simulink model "SimulareModel1"  (R2023a)
settings: Solver=VariableStepAuto  StartTime=0.0  StopTime=75.3  RelTol=1e-3
values from neighbouring files (symbols this model uses):
  Ts = 0.1    [NonLinearARXModel.mat]    (also in NonLinearHammerstein-Weiner.mat; Workspace.mat)
settings Model: Creator=petri  LastModifiedBy=petri

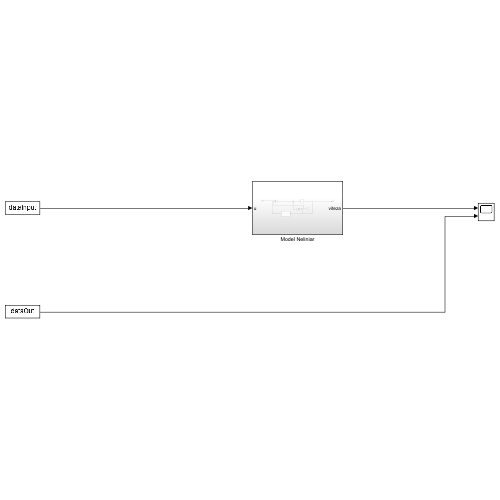
[thumbnail: Simulink's stored preview of the top-level diagram]
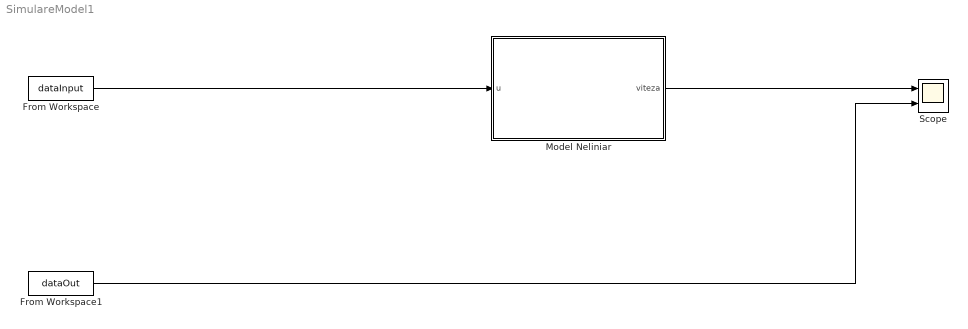
== system SimulareModel1 ==
  From Workspace : FromWorkspace  VariableName=dataInput  SampleTime=Ts
  From Workspace1 : FromWorkspace  VariableName=dataOut  SampleTime=Ts
  Model Neliniar : Subsystem
  Scope : Scope  NumInputPorts=2
  wires:
  From Workspace/1 -> Model Neliniar/1(u)
  Model Neliniar/1(viteza) -> Scope/1
  From Workspace1/1 -> Scope/2

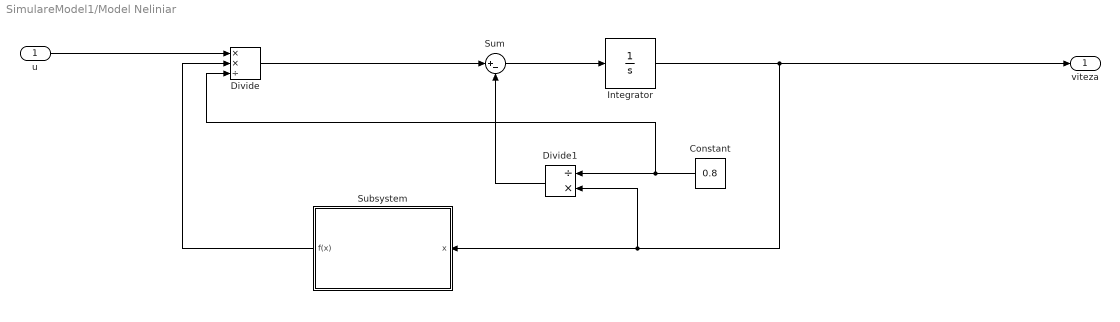
== system SimulareModel1/Model Neliniar ==
  u : Inport
  Constant : Constant  Value=0.8
  Divide : Product  Inputs=**/
  Divide1 : Product  Inputs=/*
  Integrator : Integrator
  Subsystem : Subsystem
  Sum : Sum  Inputs=|+-
  viteza : Outport
  wires:
  u/1 -> Divide/1
  Constant/1 -> Divide1/1, Divide/3
  Integrator/1 -> viteza/1, Subsystem/1(x), Divide1/2
  Sum/1 -> Integrator/1
  Divide1/1 -> Sum/2
  Divide/1 -> Sum/1
  Subsystem/1(f(x)) -> Divide/2

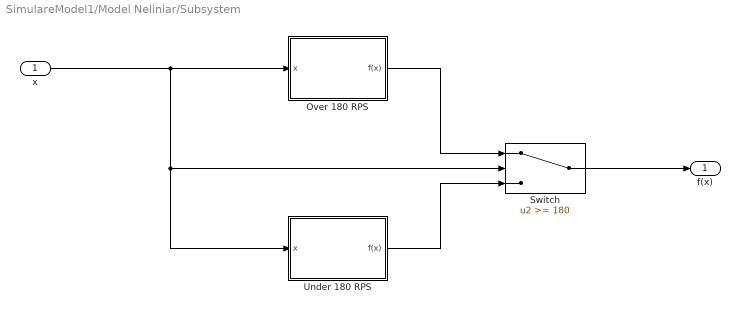
== system SimulareModel1/Model Neliniar/Subsystem ==
  x : Inport
  Over 180 RPS : Subsystem
  Switch : Switch  Threshold=180  SaturateOnIntegerOverflow=off  InputSameDT=off
  Under 180 RPS : Subsystem
  f(x) : Outport
  wires:
  x/1 -> Under 180 RPS/1(x), Switch/2, Over 180 RPS/1(x)
  Under 180 RPS/1(f(x)) -> Switch/3
  Over 180 RPS/1(f(x)) -> Switch/1
  Switch/1 -> f(x)/1

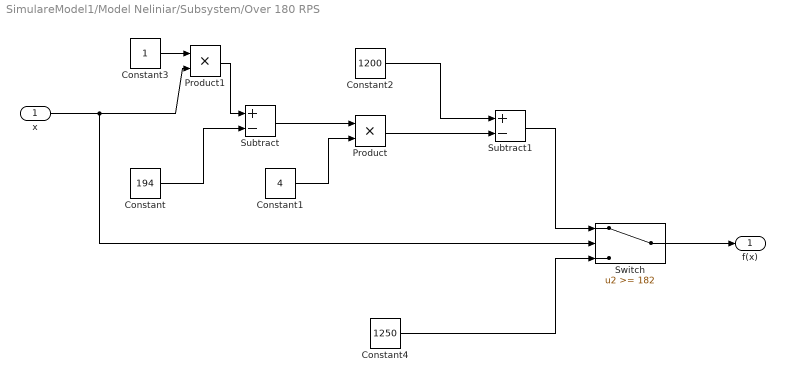
== system SimulareModel1/Model Neliniar/Subsystem/Over 180 RPS ==
  x : Inport
  Constant : Constant  Value=194  VectorParams1D=off
  Constant1 : Constant  Value=4
  Constant2 : Constant  Value=1200
  Constant3 : Constant
  Constant4 : Constant  Value=1250
  Product : Product
  Product1 : Product
  Subtract : Sum  Inputs=+-
  Subtract1 : Sum  Inputs=+-
  Switch : Switch  Threshold=182  SaturateOnIntegerOverflow=off  InputSameDT=off
  f(x) : Outport
  wires:
  x/1 -> Product1/2, Switch/2
  Product/1 -> Subtract1/2
  Constant3/1 -> Product1/1
  Constant/1 -> Subtract/2
  Subtract/1 -> Product/1
  Product1/1 -> Subtract/1
  Constant1/1 -> Product/2
  Constant2/1 -> Subtract1/1
  Constant4/1 -> Switch/3
  Subtract1/1 -> Switch/1
  Switch/1 -> f(x)/1

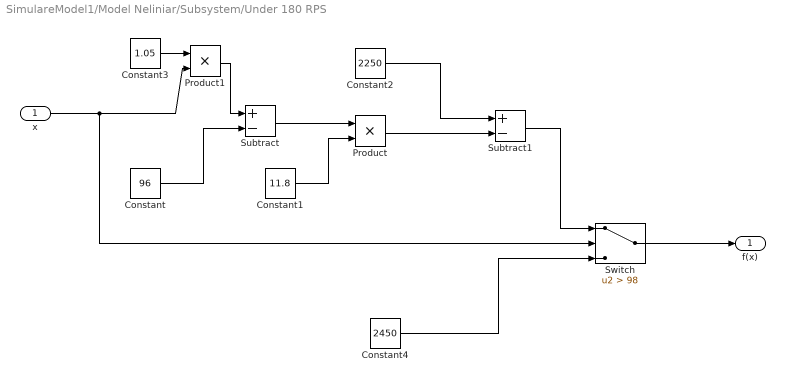
== system SimulareModel1/Model Neliniar/Subsystem/Under 180 RPS ==
  x : Inport
  Constant : Constant  Value=96
  Constant1 : Constant  Value=11.8
  Constant2 : Constant  Value=2250
  Constant3 : Constant  Value=1.05
  Constant4 : Constant  Value=2450
  Product : Product
  Product1 : Product
  Subtract : Sum  Inputs=+-
  Subtract1 : Sum  Inputs=+-
  Switch : Switch  Criteria=u2 > Threshold  Threshold=98  SaturateOnIntegerOverflow=off  InputSameDT=off
  f(x) : Outport
  wires:
  x/1 -> Product1/2, Switch/2
  Product/1 -> Subtract1/2
  Constant3/1 -> Product1/1
  Constant/1 -> Subtract/2
  Subtract/1 -> Product/1
  Product1/1 -> Subtract/1
  Constant1/1 -> Product/2
  Constant2/1 -> Subtract1/1
  Constant4/1 -> Switch/3
  Subtract1/1 -> Switch/1
  Switch/1 -> f(x)/1
